simulink library "neuromorphic_blocks"  (R2022a)
settings: Solver=VariableStepAuto  StartTime=0.0  StopTime=10.0  RelTol=1e-3
libraries: $bdroot x47, simulink x7
(part 1 of 3)
settings Model: Creator=chris  LastModifiedBy=chris

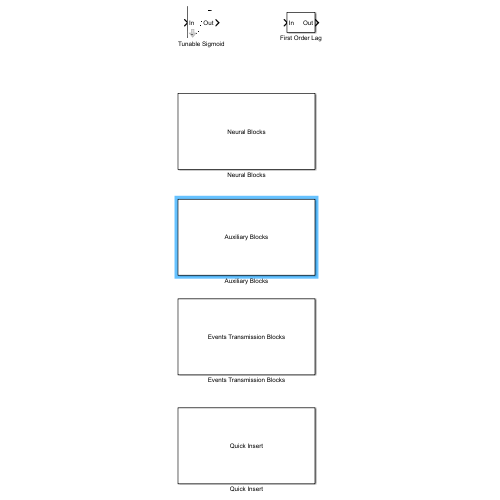
[thumbnail: Simulink's stored preview of the top-level diagram]
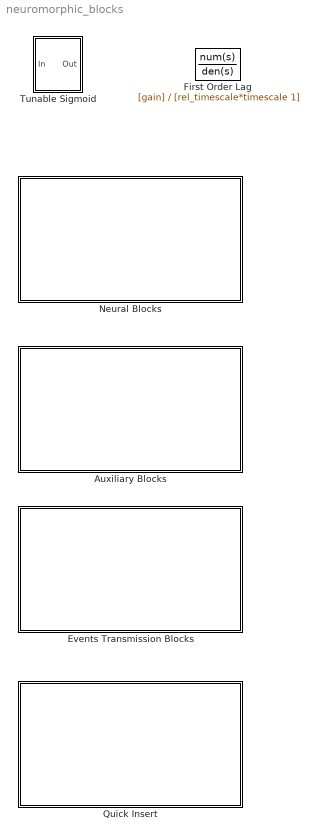
== system neuromorphic_blocks ==
  Auxiliary Blocks : Subsystem
      mask Display: disp('Auxiliary Blocks');
  Events Transmission Blocks : Subsystem
      mask Display: disp('Events Transmission Blocks');
  First Order Lag : TransferFcn  Numerator=[gain]  Denominator=[rel_timescale*timescale 1]  mask(First Order Lag){gain=1, timescale=0.004, rel_timescale=1}
      mask help: Wrapper around Low-Pass Filter block of simulink to make it consistent with other blocks in the toolbox.
      mask DialogControl gain_text Prompt: Gain
      mask DialogControl timescale_text Prompt: Timescale
      mask DialogControl rel_timescale_text Prompt: Relative Timescale
      mask Display:
      | port_label('output', 1, 'Out');
      | port_label('input', 1, 'In');
  Neural Blocks : Subsystem
      mask Display: disp('Neural Blocks');
  Quick Insert : Subsystem
      mask Display: disp("Quick Insert")
  Tunable Sigmoid : Subsystem  mask(Tunable Sigmoid){nonlinearity_type=Sigmoid, gain_source=Internal, gain=0, bias=0, slope=1}
      mask prompts: gain_source "Source"; gain "Value"; bias "Value"; slope "Value"
      mask help:
      | Sigmoid where gain can be set by external input.
      | The block can be set in Tanh or Sigmoid mode.
      mask init:
      | mask  = Simulink.Mask.get(gcb);
      | 
      |     %type_chosen = mask.getParameter('nonlinearity_type').Value;
      |     %set_param([gcb '/VSNK' ],'LabelModeActiveChoice', type_chosen);
      |     %set_param([gcb '/VSRC' ],'LabelModeActiveChoice', type_chosen);
      |     %disp(type_chosen)
      | 
      |     switch mask.getParameter('nonlinearity_type').Value
      |         case 'Sigmoid'
      |             set_param([gcb '/VSNK' ],'LabelModeActiveChoice', 'Sigmoid');
      |             set_param([gcb '/VSRC' ],'LabelModeActiveChoice', 'Sigmoid');
      |         case 'Tanh'
      |             set_param([gcb '/VSNK' ],'LabelModeActiveChoice', 'Tanh');
      |             set_param([gcb '/VSRC' ],'LabelModeActiveChoice', 'Tanh');
      |     end
      | 
      | 
      |     type = {get_param([gcb '/gain'],'BlockType')};
      |     switch mask.getParameter('gain_source').Value
      |         case 'Internal'
      |             if ismember(type, {'Inport'})
      |                 replace_block([gcb '/gain'], 'Inport', 'Constant', 'noprompt');
      |             end
      |             set_param([gcb '/gain'],'Value','gain');
      |         case 'External'
      |             if ismember(type, {'Constant'})
      |                 replace_block([gcb '/gain'], 'Constant', 'Inport', 'noprompt');
      |             end
      |     end
      mask TypeOptions nonlinearity_type: Sigmoid | Tanh
      mask TypeOptions gain_source: Internal | External
      mask Callback gain_source:
      | mask  = Simulink.Mask.get(gcb);
      |     switch mask.getParameter('gain_source').Value
      |         case 'Internal'
      |             mask.getParameter('gain').Enabled = 'on';
      |         case 'External'
      |             mask.getParameter('gain').Enabled = 'off';
      |     end
      mask DialogControl type_text Prompt: Type
      mask DialogControl gain_text Prompt: Gain
      mask DialogControl bias_text Prompt: Bias
      mask DialogControl slope_text Prompt: Slope
      mask Display:
      | mask  = Simulink.Mask.get(gcb);
      | [gain, gain_converted] = str2num(mask.getParameter('gain').Value);
      | [slope, slope_converted] = str2num(mask.getParameter('slope').Value);
      | 
      | if strcmp(mask.getParameter('gain_source').Value,'Internal') ...
      |    && gain_converted && slope_converted && gain*slope < 0
      |     image('icons/tanh_reversed.jpg');
      | else
      |     image('icons/tanh.jpg');
      | end
      | 
      | 
      | port_label('output', 1, 'Out');
      | 
      | simBlockH = get_param(gcb, 'Handle');
      | portH = find_system(simBlockH, 'LookUnderMasks', 'on', 'FollowLinks', 'on', 'SearchDepth', 1, 'BlockType', 'Inport');
      | portNames = cellstr(get_param(portH, 'Name'));
      | portNum = cellstr(get_param(portH, 'Port'));
      | for i = 1:length(portNames)
      |     if ~isempty(portNames{i})
      |         num = str2num(['uint8(' portNum{i} ')']);
      |         port_label('input', num, portNames{i});
      |     end
      | end

== system neuromorphic_blocks/Auxiliary Blocks ==
  Directional Threshold Detector : Subsystem  mask(Directional Event Generator){gain_in=-1, bias_in=0, slope_in=1, output=Events, gain_out=1, bias_out=0, slope_out=1, Iapp_base=0, V0=-1.2, dfm=0, dsp=0.5, dup=-0.5, gfm=2, gsp=4, gup=15, mfm=1, msp=1, mup=1, rel_fast=0.1, rel_membrane=0.1, rel_slow=4, timescale=0.004, tresh=0}
      mask prompts: Iapp_base "Value"; V0 "Value"; dfm "Value"; dsp "Value"; dup "Value"; gfm "Value"; gsp "Value"; gup "Value"; mfm "Value"; msp "Value"; mup "Value"; rel_fast "Value"; rel_membrane "Value"; rel_slow "Value"; timescale "Value"; tresh "Value"
      mask init:
      | mask = Simulink.Mask.get(gcb);
      | 
      |     type_V = get_param([gcb '/V'],'BlockType');
      |     type_Ev = get_param([gcb '/Ev'],'BlockType');
      |     switch mask.getParameter('output').Value
      |         case 'Events'
      |             switch type_V
      |                 case 'Outport'
      |                     replace_block([gcb '/V'], 'Outport', 'Terminator', 'noprompt')
      |             end
      |             switch type_Ev
      |                 case 'Terminator'
      |                     replace_block([gcb '/Ev'], 'Terminator', 'Outport', 'noprompt')
      |             end
      |             set_param([gcb '/Out Sigmoid'],'Commented','off')
      |         case 'Voltage'
      |             switch type_V
      |                 case 'Terminator'
      |                     replace_block([gcb '/V'], 'Terminator', 'Outport', 'noprompt')
      |             end
      |             switch type_Ev
      |                 case 'Outport'
      |                     replace_block([gcb '/Ev'], 'Outport', 'Terminator', 'noprompt')
      |             end
      |             set_param([gcb '/Out Sigmoid'],'Commented','on')
      |     end
      mask TypeOptions gain_in: In Sigmoid/gain
      mask TypeOptions bias_in: In Sigmoid/bias
      mask TypeOptions slope_in: In Sigmoid/slope
      mask TypeOptions output: Events | Voltage
      mask Callback output:
      | mask = Simulink.Mask.get(gcb);
      |     param_list = {'gain_out', 'bias_out', 'slope_out'};
      |     switch mask.getParameter('output').Value
      |         case 'Events'
      |             for param_cell = param_list
      |                 param = param_cell{1};
      |                 %mask.getParameter(param).Enabled = 'off';
      |                 mask.getParameter(param).Visible = 'off';
      |                 %mask.getDialogControl([param '_text']).Enabled = 'off';
      |                 mask.getDialogControl([param '_text']).Visible = 'off';
      |             end
      |         case 'Voltage'
      |             for param_cell = param_list
      |                 param = param_cell{1};
      |                 %mask.getParameter(param).Enabled = 'on';
      |                 mask.getParameter(param).Visible = 'on';
      |                 %mask.getDialogControl([param '_text']).Enabled = 'on';
      |                 mask.getDialogControl([param '_text']).Visible = 'on';
      |             end
      |     end
      mask TypeOptions gain_out: Out Sigmoid/gain
      mask TypeOptions bias_out: Out Sigmoid/bias
      mask TypeOptions slope_out: Out Sigmoid/slope
      mask TypeOptions Iapp_base: Rebound Neuron/Iapp_base
      mask TypeOptions V0: Rebound Neuron/V0
      mask TypeOptions dfm: Rebound Neuron/dfm
      mask TypeOptions dsp: Rebound Neuron/dsp
      mask TypeOptions dup: Rebound Neuron/dup
      mask TypeOptions gfm: Rebound Neuron/gfm
      mask TypeOptions gsp: Rebound Neuron/gsp
      mask TypeOptions gup: Rebound Neuron/gup
      mask TypeOptions mfm: Rebound Neuron/mfm
      mask TypeOptions msp: Rebound Neuron/msp
      mask TypeOptions mup: Rebound Neuron/mup
      mask TypeOptions rel_fast: Rebound Neuron/rel_fast
      mask TypeOptions rel_membrane: Rebound Neuron/rel_membrane
      mask TypeOptions rel_slow: Rebound Neuron/rel_slow
      mask TypeOptions timescale: Rebound Neuron/timescale
      mask TypeOptions tresh: Rebound Neuron/tresh
      mask DialogControl gain_in_text Prompt: Input Gain
      mask DialogControl bias_in_text Prompt: Input Bias
      mask DialogControl slope_in_text Prompt: Input Slope
      mask DialogControl output_text Prompt: Output
      mask DialogControl gain_out_text Prompt: Output Gain
      mask DialogControl bias_out_text Prompt: Output Bias
      mask DialogControl slope_out_text Prompt: Output Slope
      mask Display:
      | mask  = Simulink.Mask.get(gcb);
      | [gain_in, gain_in_converted] = str2num(mask.getParameter('gain_in').Value);
      | [slope_in, slope_in_converted] = str2num(mask.getParameter('slope_in').Value);
      | 
      | if gain_in_converted && slope_in_converted && gain_in*slope_in < 0
      |     image('icons/threshold_reversed.jpg');
      | else
      |     image('icons/threshold.jpg');
      | end
      | 
      | simBlockH = get_param(gcb, 'Handle');
      | 
      | 
      | portH = find_system(simBlockH, 'LookUnderMasks', 'on', 'FollowLinks', 'on', 'SearchDepth', 1, 'BlockType', 'Inport');
      | portNames = cellstr(get_param(portH, 'Name'));
      | portNum = cellstr(get_param(portH, 'Port'));
      | for i = 1:length(portNames)
      |     if ~isempty(portNames{i})
      |         num = str2num(['uint8(' portNum{i} ')']);
      |         port_label('input', num, portNames{i});
      |     end
      | end
      | 
      | portH = find_system(simBlockH, 'LookUnderMasks', 'on', 'FollowLinks', 'on', 'SearchDepth', 1, 'BlockType', 'Outport');
      | portNames = cellstr(get_param(portH, 'Name'));
      | portNum = cellstr(get_param(portH, 'Port'));
      | for i = 1:length(portNames)
      |     if ~isempty(portNames{i})
      |         num = str2num(['uint8(' portNum{i} ')']);
      |         port_label('output', num, portNames{i});
      |     end
      | end
  Event-Signal Multiplier : Subsystem  mask(Event Demux){symmetric_box=off, dsyn_signal_pos=0, dsyn_signal_neg=0, dsyn_signal_neg_save=0, gain_signal_pos=1, gain_signal_neg=1, gain_signal_neg_save=1, input=Events, gsyn_pos=0, gsyn_neg=0, gsyn_neg_save=0, dsyn_event_pos=0, dsyn_event_neg=0, dsyn_event_neg_save=0, gain_event_pos=1, gain_event_neg=1, gain_event_neg_save=1}
      mask prompts: symmetric_box "Differentiate positive and negative parameters"; dsyn_signal_pos "Value"; dsyn_signal_neg "Neg"; dsyn_signal_neg_save "Save"; gain_signal_pos "Value"; gain_signal_neg "Neg"; gain_signal_neg_save "Save"; gsyn_pos "Value"; gsyn_neg "Neg"; gsyn_neg_save "Save"; dsyn_event_pos "Value"; dsyn_event_neg "Neg"; dsyn_event_neg_save "Save"; gain_event_pos "Value"; gain_event_neg "Neg"; gain_event_neg_save "Save"
      mask init:
      | mask  = Simulink.Mask.get(gcb);
      |     switch mask.getParameter('input').Value
      |         case 'Events'
      |             %set_param([gcb '/VSNK_ev' ],'LabelModeActiveChoice', 'Events');
      |             %set_param([gcb '/VSNK_s' ],'LabelModeActiveChoice', 'Events');
      |             %set_param([gcb '/VSRC' ],'LabelModeActiveChoice', 'Events');
      |             set_param([gcb '/VSub' ],'LabelModeActiveChoice', 'Events');
      |             %mask.getPortConstraint('inout_main_type').Rule.DataType = {'boolean'};
      |             try
      |                 set_param([gcb '/V'], 'Name', 'Ev');
      |                 set_param([gcb '/V+'], 'Name', 'Ev+');
      |                 set_param([gcb '/V-'], 'Name', 'Ev-');
      |             catch E
      |             end
      |         case 'Voltage'
      |             %set_param([gcb '/VSNK_ev' ],'LabelModeActiveChoice', 'Voltage');
      |             %set_param([gcb '/VSNK_s' ],'LabelModeActiveChoice', 'Voltage');
      |             %set_param([gcb '/VSRC' ],'LabelModeActiveChoice', 'Voltage');
      |             set_param([gcb '/VSub' ],'LabelModeActiveChoice', 'Voltage');
      |             %mask.getPortConstraint('inout_main_type').Rule.DataType = {'double'; 'single'; 'int8'; 'uint8'; 'int16'; 'uint16'; 'int32'; 'uint32'};
      |             try
      |                 set_param([gcb '/Ev'], 'Name', 'V');
      |                 set_param([gcb '/Ev+'], 'Name', 'V+');
      |                 set_param([gcb '/Ev-'], 'Name', 'V-');
      |             catch E
      |             end
      |     end
      | 
      |     suffix_list = {'gsyn', 'dsyn_event', 'gain_event', 'dsyn_signal', 'gain_signal'};
      |     switch mask.getParameter('symmetric_box').Value
      |         case 'off'
      |             for suffix_cell = suffix_list
      |                 suffix = suffix_cell{1};
      |                 mask.getParameter([suffix '_neg']).Value = mask.getParameter([suffix '_pos']).Value;
      |             end
      |         case 'on'
      |             for suffix_cell = suffix_list
      |                 suffix = suffix_cell{1};
      |                 mask.getParameter([suffix '_neg']).Value = mask.getParameter([suffix '_neg_save']).Value;
      |             end
      |     end
      mask Callback symmetric_box:
      | mask  = Simulink.Mask.get(gcb);
      |     switch mask.getParameter('input').Value
      |         case 'Events'
      |             suffix_list = {'dsyn_signal', 'gain_signal'};
      |         case 'Voltage'
      |             suffix_list = {'dsyn_signal', 'gain_signal', 'gsyn', 'dsyn_event', 'gain_event'};
      |     end
      | 
      |     switch mask.getParameter('symmetric_box').Value
      |         case 'on'
      |             for suffix_cell = suffix_list
      |                 suffix = suffix_cell{1};
      |                 %mask.getParameter([suffix '_neg']).Hidden = 'off';
      |                 %mask.getParameter([suffix '_neg_save']).ReadOnly = 'off';
      |                 mask.getParameter([suffix '_neg']).Value = mask.getParameter([suffix '_neg_save']).Value;
      |                 %mask.getParameter([suffix '_neg']).Enabled = 'on';
      |                 mask.getParameter([suffix '_neg']).Visible = 'on';
      |                 mask.getParameter([suffix '_pos']).Prompt = 'Pos';
      |             end
      |         case 'off'
      |             for suffix_cell = suffix_list
      |                 suffix = suffix_cell{1};
      |                 %mask.getParameter([suffix '_neg_save']).Value = mask.getParameter([suffix '_neg']).Value;
      |                 %mask.getParameter([suffix '_neg_save']).ReadOnly = 'on';
      |                 %mask.getParameter([suffix '_neg']).Enabled = 'off';
      |                 mask.getParameter([suffix '_neg']).Visible = 'off';
      |                 mask.getParameter([suffix '_pos']).Prompt = 'Value';
      |                 %mask.getParameter([suffix '_neg']).Value = mask.getParameter([suffix '_pos']).Value;
      |                 %mask.getParameter([suffix '_neg']).Hidden = 'on';
      |             end
      |     end
      mask Callback dsyn_signal_neg:
      | suffix = 'dsyn_signal';
      |     mask  = Simulink.Mask.get(gcb);
      |     switch mask.getParameter('symmetric_box').Value
      |         case 'on'
      |              mask.getParameter([suffix '_neg_save']).Value = mask.getParameter([suffix '_neg']).Value;
      |     end
      mask Callback gain_signal_neg:
      | suffix = 'gain_signal';
      |     mask  = Simulink.Mask.get(gcb);
      |     switch mask.getParameter('symmetric_box').Value
      |         case 'on'
      |              mask.getParameter([suffix '_neg_save']).Value = mask.getParameter([suffix '_neg']).Value;
      |     end
      mask TypeOptions input: Events | Voltage
      mask Callback input:
      | mask = Simulink.Mask.get(gcb);
      |     suffix_list = {'gsyn', 'dsyn_event', 'gain_event'};
      |     switch mask.getParameter('input').Value
      |         case 'Events'
      |             for suffix_cell = suffix_list
      |                 suffix = suffix_cell{1};
      |                 %mask.getParameter([suffix '_pos']).Enabled = 'off';
      |                 mask.getParameter([suffix '_pos']).Visible = 'off';
      |                 %mask.getParameter([suffix '_neg']).Enabled = 'off';
      |                 mask.getParameter([suffix '_neg']).Visible = 'off';
      |                 %mask.getDialogControl([suffix '_text']).Enabled = 'off';
      |                 mask.getDialogControl([suffix '_text']).Visible = 'off';
      |             end
      |         case 'Voltage'
      |             switch mask.getParameter('symmetric_box').Value
      |                 case 'on'
      |                     enable_neg = true;
      |                 case 'off'
      |                     enable_neg = false;
      |             end
      |             for suffix_cell = suffix_list
      |                 suffix = suffix_cell{1};
      |                 %mask.getParameter([suffix '_pos']).Enabled = 'on';
      |                 mask.getParameter([suffix '_pos']).Visible = 'on';
      |                 %mask.getDialogControl([suffix '_text']).Enabled = 'on';
      |                 mask.getDialogControl([suffix '_text']).Visible = 'on';
      |                 if enable_neg
      |                     %mask.getParameter([suffix '_neg']).Enabled = 'on';
      |                     mask.getParameter([suffix '_neg']).Visible = 'on';
      |                 end
      |             end
      |     end
      mask Callback gsyn_neg:
      | suffix = 'gsyn';
      |     mask  = Simulink.Mask.get(gcb);
      |     switch mask.getParameter('symmetric_box').Value
      |         case 'on'
      |              mask.getParameter([suffix '_neg_save']).Value = mask.getParameter([suffix '_neg']).Value;
      |     end
      mask Callback dsyn_event_neg:
      | suffix = 'dsyn_event';
      |     mask  = Simulink.Mask.get(gcb);
      |     switch mask.getParameter('symmetric_box').Value
      |         case 'on'
      |              mask.getParameter([suffix '_neg_save']).Value = mask.getParameter([suffix '_neg']).Value;
      |     end
      mask Callback gain_event_neg:
      | suffix = 'gain_event';
      |     mask  = Simulink.Mask.get(gcb);
      |     switch mask.getParameter('symmetric_box').Value
      |         case 'on'
      |              mask.getParameter([suffix '_neg_save']).Value = mask.getParameter([suffix '_neg']).Value;
      |     end
      mask DialogControl dsyn_signal_text Prompt: Signal Bias
      mask DialogControl gain_signal_text Prompt: Signal Slope
      mask DialogControl input_text Prompt: Input-Output Type
      mask DialogControl gsyn_text Prompt: Event Gain
      mask DialogControl dsyn_event_text Prompt: Event Bias
      mask DialogControl gain_event_text Prompt: Event Slope
      mask Display:
      | simBlockH = get_param(gcb, 'Handle');
      | 
      | image("icons/event_mul.jpg")
      | 
      | portH = find_system(simBlockH, 'LookUnderMasks', 'on', 'FollowLinks', 'on', 'SearchDepth', 1, 'BlockType', 'Inport');
      | portNames = cellstr(get_param(portH, 'Name'));
      | portNum = cellstr(get_param(portH, 'Port'));
      | for i = 1:length(portNames)
      |     if ~isempty(portNames{i})
      |         num = str2num(['uint8(' portNum{i} ')']);
      |         port_label('input', num, portNames{i});
      |     end
      | end
      | 
      | portH = find_system(simBlockH, 'LookUnderMasks', 'on', 'FollowLinks', 'on', 'SearchDepth', 1, 'BlockType', 'Outport');
      | portNames = cellstr(get_param(portH, 'Name'));
      | portNum = cellstr(get_param(portH, 'Port'));
      | for i = 1:length(portNames)
      |     if ~isempty(portNames{i})
      |         num = str2num(['uint8(' portNum{i} ')']);
      |         port_label('output', num, portNames{i});
      |     end
      | end
  Event-Signal Selector : Subsystem  mask(Event Mux){symmetric_box=off, dsyn_signal_pos=0, dsyn_signal_neg=0, dsyn_signal_neg_save=0, gain_signal_pos=1, gain_signal_neg=1, gain_signal_neg_save=1, input=Events, gsyn_pos=0, gsyn_neg=0, gsyn_neg_save=0, dsyn_event_pos=0, dsyn_event_neg=0, dsyn_event_neg_save=0, gain_event_pos=1, gain_event_neg=1, gain_event_neg_save=1}
      mask prompts: symmetric_box "Differentiate positive and negative parameters"; dsyn_signal_pos "Value"; dsyn_signal_neg "Neg"; dsyn_signal_neg_save "Save"; gain_signal_pos "Value"; gain_signal_neg "Neg"; gain_signal_neg_save "Save"; gsyn_pos "Value"; gsyn_neg "Neg"; gsyn_neg_save "Save"; dsyn_event_pos "Value"; dsyn_event_neg "Neg"; dsyn_event_neg_save "Save"; gain_event_pos "Value"; gain_event_neg "Neg"; gain_event_neg_save "Save"
      mask init: same as neuromorphic_blocks/Auxiliary Blocks/Event-Signal Multiplier
      mask Callback symmetric_box:
      | mask  = Simulink.Mask.get(gcb);
      |     switch mask.getParameter('input').Value
      |         case 'Events'
      |             suffix_list = {'dsyn_signal', 'gain_signal'};
      |         case 'Voltage'
      |             suffix_list = {'dsyn_signal', 'gain_signal', 'gsyn', 'dsyn_event', 'gain_event'};
      |     end
      | 
      |     switch mask.getParameter('symmetric_box').Value
      |         case 'on'
      |             for suffix_cell = suffix_list
      |                 suffix = suffix_cell{1};
      |                 %mask.getParameter([suffix '_neg']).Hidden = 'off';
      |                 %mask.getParameter([suffix '_neg_save']).ReadOnly = 'off';
      |                 mask.getParameter([suffix '_neg']).Value = mask.getParameter([suffix '_neg_save']).Value;
      |                 %mask.getParameter([suffix '_neg']).Enabled = 'on';
      |                 mask.getParameter([suffix '_neg']).Visible = 'on';
      |                 mask.getParameter([suffix '_pos']).Prompt = 'Pos';
      |             end
      |         case 'off'
      |             for suffix_cell = suffix_list
      |                 suffix = suffix_cell{1};
      |                 %mask.getParameter([suffix '_neg_save']).Value = mask.getParameter([suffix '_neg']).Value;
      |                 %mask.getParameter([suffix '_neg_save']).ReadOnly = 'on';
      |                 %mask.getParameter([suffix '_neg']).Enabled = 'off';
      |                 mask.getParameter([suffix '_neg']).Visible = 'off';
      |                 mask.getParameter([suffix '_pos']).Prompt = 'Value';
      |                 %mask.getParameter([suffix '_neg']).Value = mask.getParameter([suffix '_pos']).Value;
      |                 %mask.getParameter([suffix '_neg']).Hidden = 'on';
      |             end
      |     end
      mask Callback dsyn_signal_neg:
      | suffix = 'dsyn_signal';
      |     mask  = Simulink.Mask.get(gcb);
      |     switch mask.getParameter('symmetric_box').Value
      |         case 'on'
      |              mask.getParameter([suffix '_neg_save']).Value = mask.getParameter([suffix '_neg']).Value;
      |     end
      mask Callback gain_signal_neg:
      | suffix = 'gain_signal';
      |     mask  = Simulink.Mask.get(gcb);
      |     switch mask.getParameter('symmetric_box').Value
      |         case 'on'
      |              mask.getParameter([suffix '_neg_save']).Value = mask.getParameter([suffix '_neg']).Value;
      |     end
      mask TypeOptions input: Events | Voltage
      mask Callback input:
      | mask = Simulink.Mask.get(gcb);
      |     suffix_list = {'gsyn', 'dsyn_event', 'gain_event'};
      |     switch mask.getParameter('input').Value
      |         case 'Events'
      |             for suffix_cell = suffix_list
      |                 suffix = suffix_cell{1};
      |                 %mask.getParameter([suffix '_pos']).Enabled = 'off';
      |                 mask.getParameter([suffix '_pos']).Visible = 'off';
      |                 %mask.getParameter([suffix '_neg']).Enabled = 'off';
      |                 mask.getParameter([suffix '_neg']).Visible = 'off';
      |                 %mask.getDialogControl([suffix '_text']).Enabled = 'off';
      |                 mask.getDialogControl([suffix '_text']).Visible = 'off';
      |             end
      |         case 'Voltage'
      |             switch mask.getParameter('symmetric_box').Value
      |                 case 'on'
      |                     enable_neg = true;
      |                 case 'off'
      |                     enable_neg = false;
      |             end
      |             for suffix_cell = suffix_list
      |                 suffix = suffix_cell{1};
      |                 %mask.getParameter([suffix '_pos']).Enabled = 'on';
      |                 mask.getParameter([suffix '_pos']).Visible = 'on';
      |                 %mask.getDialogControl([suffix '_text']).Enabled = 'on';
      |                 mask.getDialogControl([suffix '_text']).Visible = 'on';
      |                 if enable_neg
      |                     %mask.getParameter([suffix '_neg']).Enabled = 'on';
      |                     mask.getParameter([suffix '_neg']).Visible = 'on';
      |                 end
      |             end
      |     end
      mask Callback gsyn_neg:
      | suffix = 'gsyn';
      |     mask  = Simulink.Mask.get(gcb);
      |     switch mask.getParameter('symmetric_box').Value
      |         case 'on'
      |              mask.getParameter([suffix '_neg_save']).Value = mask.getParameter([suffix '_neg']).Value;
      |     end
      mask Callback dsyn_event_neg:
      | suffix = 'dsyn_event';
      |     mask  = Simulink.Mask.get(gcb);
      |     switch mask.getParameter('symmetric_box').Value
      |         case 'on'
      |              mask.getParameter([suffix '_neg_save']).Value = mask.getParameter([suffix '_neg']).Value;
      |     end
      mask Callback gain_event_neg:
      | suffix = 'gain_event';
      |     mask  = Simulink.Mask.get(gcb);
      |     switch mask.getParameter('symmetric_box').Value
      |         case 'on'
      |              mask.getParameter([suffix '_neg_save']).Value = mask.getParameter([suffix '_neg']).Value;
      |     end
      mask DialogControl dsyn_signal_text Prompt: Signal Bias
      mask DialogControl gain_signal_text Prompt: Signal Slope
      mask DialogControl input_text Prompt: Input-Output Type
      mask DialogControl gsyn_text Prompt: Event Gain
      mask DialogControl dsyn_event_text Prompt: Event Bias
      mask DialogControl gain_event_text Prompt: Event Slope
      mask Display:
      | simBlockH = get_param(gcb, 'Handle');
      | 
      | 
      | portH = find_system(simBlockH, 'LookUnderMasks', 'on', 'FollowLinks', 'on', 'SearchDepth', 1, 'BlockType', 'Inport');
      | portNames = cellstr(get_param(portH, 'Name'));
      | portNum = cellstr(get_param(portH, 'Port'));
      | for i = 1:length(portNames)
      |     if ~isempty(portNames{i})
      |         num = str2num(['uint8(' portNum{i} ')']);
      |         port_label('input', num, portNames{i});
      |     end
      | end
      | 
      | portH = find_system(simBlockH, 'LookUnderMasks', 'on', 'FollowLinks', 'on', 'SearchDepth', 1, 'BlockType', 'Outport');
      | portNames = cellstr(get_param(portH, 'Name'));
      | portNum = cellstr(get_param(portH, 'Port'));
      | for i = 1:length(portNames)
      |     if ~isempty(portNames{i})
      |         num = str2num(['uint8(' portNum{i} ')']);
      |         port_label('output', num, portNames{i});
      |     end
      | end
  Event-Triggered Relay : Subsystem  mask(Bistable System){gsyn_out=0, dsyn_out=0, msyn_out=0, gsyn_pos_source=Internal, gsyn_pos=0, gsyn_neg_source=Internal, gsyn_neg=0, timescale=0.004, rel_timescale=1000, input=Events, dsyn_pos=0, dsyn_neg=0, msyn_pos=1, msyn_neg=1}
      mask prompts: gsyn_out "Value"; dsyn_out "Value"; msyn_out "Value"; gsyn_pos_source "Source"; gsyn_pos "Value"; gsyn_neg_source "Source"; gsyn_neg "Value"; timescale "Value"; rel_timescale "Value"; dsyn_pos "Value"; dsyn_neg "Value"; msyn_pos "Value"; msyn_neg "Value"
      mask init:
      | mask  = Simulink.Mask.get(gcb);
      | 
      |     switch mask.getParameter('input').Value
      |         case 'Events'
      |             set_param([gcb '/VSNK_pos'],'LabelModeActiveChoice', 'Events');
      |             set_param([gcb '/VSRC_pos'],'LabelModeActiveChoice', 'Events');
      |             set_param([gcb '/VSNK_neg'],'LabelModeActiveChoice', 'Events');
      |             set_param([gcb '/VSRC_neg'],'LabelModeActiveChoice', 'Events');
      |             %mask.getPortConstraint('in_main_type').Rule.DataType = {'boolean'};
      |             try
      |                 set_param([gcb '/V+'], 'Name', 'Ev+');
      |                 set_param([gcb '/V-'], 'Name', 'Ev-');
      |             catch E
      |             end
      |         case 'Voltage'
      |             set_param([gcb '/VSNK_pos'],'LabelModeActiveChoice', 'Voltage');
      |             set_param([gcb '/VSRC_pos'],'LabelModeActiveChoice', 'Voltage');
      |             set_param([gcb '/VSNK_neg'],'LabelModeActiveChoice', 'Voltage');
      |             set_param([gcb '/VSRC_neg'],'LabelModeActiveChoice', 'Voltage');
      |             %mask.getPortConstraint('in_main_type').Rule.DataType = {'double'; 'single'; 'int8'; 'uint8'; 'int16'; 'uint16'; 'int32'; 'uint32'};
      |             try
      |                 set_param([gcb '/Ev+'], 'Name', 'V+');
      |                 set_param([gcb '/Ev-'], 'Name', 'V-');
      |             catch E
      |             end
      |     end
      | 
      |     switch mask.getParameter('gsyn_pos_source').Value
      |         case 'Internal'
      |             replace_block([gcb '/gsyn_pos'], 'Inport', 'Constant', 'noprompt');
      |             set_param([gcb '/gsyn_pos'],'Value','gsyn_pos');
      |             if strcmp('0', mask.getParameter(['gsyn_pos']).Value)
      |                 set_param([gcb '/Isyn_pos'],'Commented','on')
      |             else
      |                 set_param([gcb '/Isyn_pos'],'Commented','off')
      |             end
      |         case 'External'
      |             set_param([gcb '/Isyn_pos'],'Commented','on')
      |             replace_block([gcb '/gsyn_pos'], 'Constant', 'Inport', 'noprompt');
      |     end
      | 
      |     switch mask.getParameter('gsyn_neg_source').Value
      |         case 'Internal'
      |             replace_block([gcb '/gsyn_neg'], 'Inport', 'Constant', 'noprompt');
      |             set_param([gcb '/gsyn_neg'],'Value','gsyn_neg');
      |             if strcmp('0', mask.getParameter(['gsyn_neg']).Value)
      |                 set_param([gcb '/Isyn_neg'],'Commented','on')
      |             else
      |                 set_param([gcb '/Isyn_neg'],'Commented','off')
      |             end
      |         case 'External'
      |             set_param([gcb '/Isyn_neg'],'Commented','on')
      |             replace_block([gcb '/gsyn_neg'], 'Constant', 'Inport', 'noprompt');
      |     end
      mask TypeOptions gsyn_pos_source: Internal | External
      mask Callback gsyn_pos_source:
      | mask  = Simulink.Mask.get(gcb);
      |     switch mask.getParameter('gsyn_pos_source').Value
      |         case 'Internal'
      |             mask.getParameter('gsyn_pos').Enabled = 'on';
      |         case 'External'
      |             mask.getParameter('gsyn_pos').Enabled = 'off';
      |     end
      mask TypeOptions gsyn_neg_source: Internal | External
      mask Callback gsyn_neg_source:
      | mask  = Simulink.Mask.get(gcb);
      |     switch mask.getParameter('gsyn_neg_source').Value
      |         case 'Internal'
      |             mask.getParameter('gsyn_neg').Enabled = 'on';
      |         case 'External'
      |             mask.getParameter('gsyn_neg').Enabled = 'off';
      |     end
      mask TypeOptions input: Events | Voltage
      mask Callback input:
      | mask = Simulink.Mask.get(gcb);
      |     switch mask.getParameter('input').Value
      |         case 'Events'
      |             mask.getParameter('dsyn_pos').Enabled = 'off';
      |             mask.getParameter('dsyn_pos').Visible = 'off';
      |             mask.getDialogControl('dsyn_pos_text').Enabled = 'off';
      |             mask.getDialogControl('dsyn_pos_text').Visible = 'off';
      |             mask.getParameter('dsyn_neg').Enabled = 'off';
      |             mask.getParameter('dsyn_neg').Visible = 'off';
      |             mask.getDialogControl('dsyn_neg_text').Enabled = 'off';
      |             mask.getDialogControl('dsyn_neg_text').Visible = 'off';
      |             mask.getParameter('msyn_pos').Enabled = 'off';
      |             mask.getParameter('msyn_pos').Visible = 'off';
      |             mask.getDialogControl('msyn_pos_text').Enabled = 'off';
      |             mask.getDialogControl('msyn_pos_text').Visible = 'off';
      |             mask.getParameter('msyn_neg').Enabled = 'off';
      |             mask.getParameter('msyn_neg').Visible = 'off';
      |             mask.getDialogControl('msyn_neg_text').Enabled = 'off';
      |             mask.getDialogControl('msyn_neg_text').Visible = 'off';
      |         case 'Voltage'
      |             mask.getParameter('dsyn_pos').Enabled = 'on';
      |             mask.getParameter('dsyn_pos').Visible = 'on';
      |             mask.getDialogControl('dsyn_pos_text').Enabled = 'on';
      |             mask.getDialogControl('dsyn_pos_text').Visible = 'on';
      |             mask.getParameter('dsyn_neg').Enabled = 'on';
      |             mask.getParameter('dsyn_neg').Visible = 'on';
      |             mask.getDialogControl('dsyn_neg_text').Enabled = 'on';
      |             mask.getDialogControl('dsyn_neg_text').Visible = 'on';
      |             mask.getParameter('msyn_pos').Enabled = 'on';
      |             mask.getParameter('msyn_pos').Visible = 'on';
      |             mask.getDialogControl('msyn_pos_text').Enabled = 'on';
      |             mask.getDialogControl('msyn_pos_text').Visible = 'on';
      |             mask.getParameter('msyn_neg').Enabled = 'on';
      |             mask.getParameter('msyn_neg').Visible = 'on';
      |             mask.getDialogControl('msyn_neg_text').Enabled = 'on';
      |             mask.getDialogControl('msyn_neg_text').Visible = 'on';
      |     end
      mask DialogControl gsyn_out_text Prompt: Feedback Gain
      mask DialogControl dsyn_out_text Prompt: Feedback Bias
      mask DialogControl msyn_out_text Prompt: Feedback Slope
      mask DialogControl gsyn_pos_text Prompt: Positive Event Conductance
      mask DialogControl gsyn_neg_text Prompt: Negative Event Conductance
      mask DialogControl timescale_text Prompt: Timescale
      mask DialogControl rel_timescale_text Prompt: Relative Timescale
      mask DialogControl input_text Prompt: Input Type
      mask DialogControl dsyn_pos_text Prompt: Positive Event Bias
      mask DialogControl dsyn_neg_text Prompt: Negative Event Bias
      mask DialogControl msyn_pos_text Prompt: Positive Event Gain
      mask DialogControl msyn_neg_text Prompt: Negative Event Gain
      mask Display:
      | image('icons/bistable.jpg');
      | 
      | port_label('output', 1, 's');
      | 
      | simBlockH = get_param(gcb, 'Handle');
      | portH = find_system(simBlockH, 'LookUnderMasks', 'on', 'FollowLinks', 'on', 'SearchDepth', 1, 'BlockType', 'Inport');
      | portNames = cellstr(get_param(portH, 'Name'));
      | portNum = cellstr(get_param(portH, 'Port'));
      | for i = 1:length(portNames)
      |     if ~isempty(portNames{i})
      |         num = str2num(['uint8(' portNum{i} ')']);
      |         port_label('input', num, portNames{i});
      |     end
      | end
  Noise on Signal : Subsystem  mask(Noise on Signal){noise_pwr=0, timescale=0.004, rel_timescale=1, seed=-1, seed_mem=randi([0, 100000])}
      mask prompts: noise_pwr "Value"; timescale "Value"; rel_timescale "Value"; seed "Value"
      mask init:
      | mask  = Simulink.Mask.get(gcb);
      |     switch mask.getParameter('seed').Value
      |         case '-1'
      |             mask.getParameter('seed_mem').Value = 'randi([0, 100000])';
      |         otherwise
      |             mask.getParameter('seed_mem').Value = mask.getParameter('seed').Value;
      |     end
      mask DialogControl noise_pwr_text Prompt: Noise Power
      mask DialogControl timescale_text Prompt: Timescale
      mask DialogControl rel_timescale_text Prompt: Relative Timescale
      mask DialogControl seed_text Prompt: Seed (-1 for random seed)
      mask Display:
      | xscale = 0.8;
      | yscale = 0.8;
      | 
      | r = [-0.4326
      |    -1.6656
      |     0.1253
      |     0.2877
      |    -1.1465
      |     1.1909
      |     1.1892
      |    -0.0376
      |     0.3273
      |     0.1746
      |    -0.1867
      |     0.7258]';
      | 
      | r2 = repelem(r,2);
      | r3 = r2 - min(r2);
      | r4 = r3/max(r3);
      | r5 = r4*yscale + (1-yscale)/2;
      | 
      | 
      | t = [1 repelem(2:12,2) 13];
      | t2 = t - min(t);
      | t3 = t2/max(t2);
      | t4 = t3*xscale + (1-xscale)/2;
      | 
      | 
      | plot(t4, r5);

== system neuromorphic_blocks/Events Transmission Blocks ==
  Continuous to Event : Subsystem  mask(Continuous to Event){thresh=0}
      mask prompts: thresh "Value"
      mask DialogControl thresh_text Prompt: Threshold
      mask Display:
      | port_label('output', 1, 'Out');
      | port_label('input', 1, 'In');
  Event Loss : Subsystem  mask(Event Loss){loss_prob=0, seed=-1, seed_mem=randi([0, 100000])}
      mask prompts: loss_prob "Value"; seed "Value"
      mask init: same as neuromorphic_blocks/Auxiliary Blocks/Noise on Signal
      mask DialogControl loss_prob_text Prompt: Probability of lost event
      mask DialogControl seed_text Prompt: Seed (-1 for random seed)
      mask Display:
      | port_label('output', 1, 'Out');
      | port_label('input', 1, 'In');
  Event to Continuous : Subsystem  mask(Event to Continuous){gain=0}
      mask prompts: gain "Value"
      mask DialogControl gain_text Prompt: Event gain
      mask Display:
      | port_label('output', 1, 'Out');
      | port_label('input', 1, 'In');
  Event to Fixed Width Pulse : Subsystem  mask(Event to Fixed Width Pulse){pulse_width=0}
      mask prompts: pulse_width "Value"
      mask DialogControl pulse_width_text Prompt: Pulse Width
      mask Display:
      | port_label('output', 1, 'Out');
      | port_label('input', 1, 'In');
